simulink model "control"  (R2023a)
settings: Solver=ode4  StartTime=0.0  StopTime=10.0  FixedStep=dt  RelTol=1e-3
undefined symbols (not defined in the file): dt
settings Model: Creator=hugobuurmeijer  LastModifiedBy=hugobuurmeijer

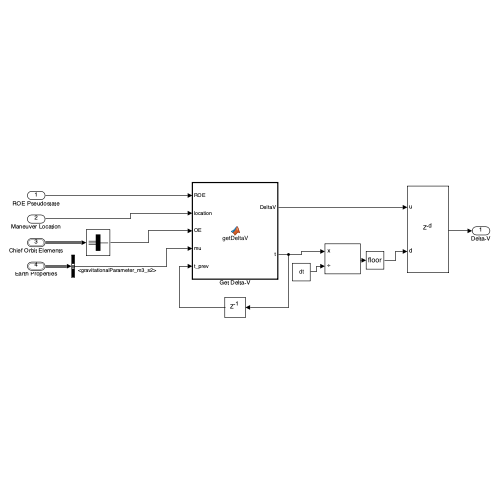
[thumbnail: Simulink's stored preview of the top-level diagram]
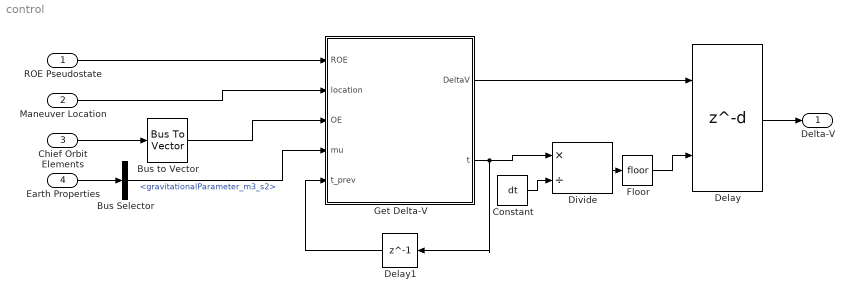
== system control ==
  ROE Pseudostate : Inport  PortDimensions=6
  Maneuver Location : Inport  Port=2  PortDimensions=50
  Chief Orbit Elements : Inport  Port=3  OutDataTypeStr=Bus: meanOrbitElements
  Earth Properties : Inport  Port=4  OutDataTypeStr=Bus: earthProperties
  Bus Selector : BusSelector  OutputSignals=gravitationalParameter_m3_s2
  Bus to Vector : BusToVector
  Constant : Constant  Value=dt
  Delay : Delay  DelayLengthSource=Input port
      settings: InputPortMap=u0,p1
  Delay1 : Delay  DelayLength=1
  Divide : Product  Inputs=*/
  Floor : Rounding
  Get Delta-V : MATLAB Function  TreatAsAtomicUnit=on
  Delta-V : Outport
  wires:
  ROE Pseudostate/1 -> Get Delta-V/1(ROE)
  Maneuver Location/1 -> Get Delta-V/2(location)
  Chief Orbit Elements/1 -> Bus to Vector/1
  Earth Properties/1 -> Bus Selector/1
  Bus to Vector/1 -> Get Delta-V/3(OE)
  Bus Selector/1 -> Get Delta-V/4(mu)  "<gravitationalParameter_m3_s2>"
  Get Delta-V/1(DeltaV) -> Delay/1
  Get Delta-V/2(t) -> Delay1/1, Divide/1
  Constant/1 -> Divide/2
  Divide/1 -> Floor/1
  Floor/1 -> Delay/2
  Delay/1 -> Delta-V/1
  Delay1/1 -> Get Delta-V/5(t_prev)

== matlab function control/Get Delta-V ==
  data: ROE input; DeltaV output; location input; OE input; mu input; t output; t_prev input
function [DeltaV,t] = getDeltaV(ROE,location,OE,mu,t_prev)
[DeltaV,t] = getDeltaV(ROE,location,OE,mu,t_prev);
end
